simulink model "OutputMVA"  (Simulink 8.7)
settings: Solver=ode45  StartTime=0.0  StopTime=10.0  RelTol=1e-3
undefined symbols (not defined in the file or in its folder): sMP
(part 1 of 3)
settings Model: Creator=rafrey5  LastModifiedBy=hillenb
settings DataIOCC: SignalLoggingSaveFormat=ModelDataLogs
settings OptimizationCC: ExpressionDepthLimit=2147483647
settings DebuggingCC: SolverPrmCheckMsg=warning  FcnCallInpInsideContextMsg=UseLocalSettings  StateNameClashWarn=warning
settings GRTTargetCC: CombineOutputUpdateFcns=off  GRTInterface=on
settings ConfigComp: CovSFcnEnable=off

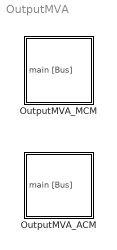
== system OutputMVA ==
  OutputMVA_ACM : Subsystem
      settings: CopyFcn=spsBusSelectorCleanup(gcb,sMP)
  OutputMVA_MCM : Subsystem
      settings: CopyFcn=spsBusSelectorCleanup(gcb,sMP)

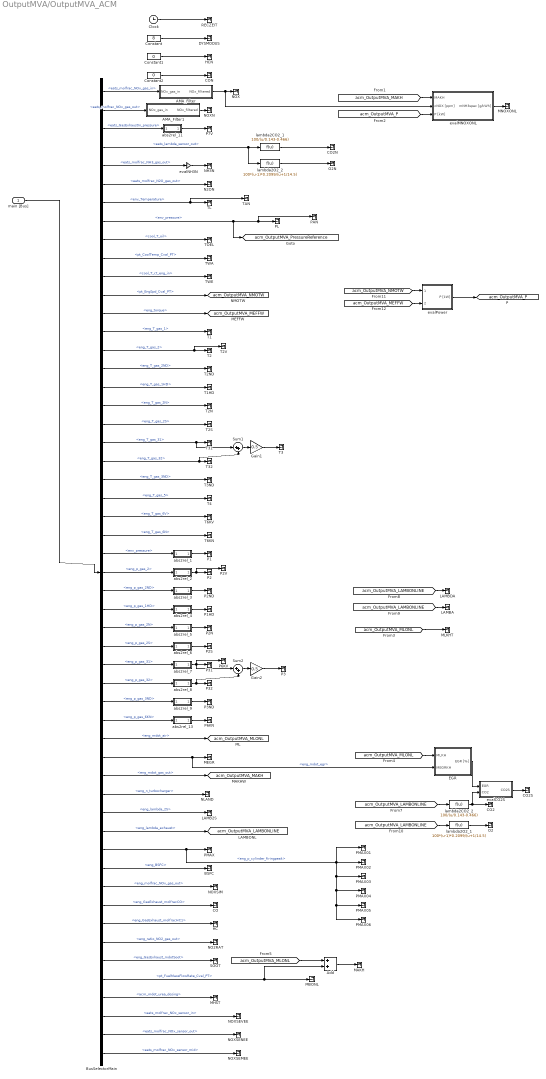
== system OutputMVA/OutputMVA_ACM ==
  main [Bus] : Inport
  AMA_Filter : Subsystem
  AMA_Filter1 : Subsystem
  Add : Sum
  BSFC : Terminator
  BusSelectorMain : BusSelector  OutputSignals=info [Bus].eats_molfrac_NOx_gas_in,info [Bus].eats_molfrac_NOx_gas_out,physics [Bus].eats_GasExhaustIn_pressure,sensor [Bus].eats_lambda_sensor_out,info [Bus].eats_molfrac_NH3_gas_out,info [Bus].eats_molfrac_N2O_gas_out,boundary [Bus].env_Temperature,boundary [Bus].env_pressure,sensor [Bus].cool_T_oil,control [Bus].pt_CoolTemp_Cval_PT,sensor [Bus].cool_T_ct_eng_in,control [Bus].pt_EngSpd_Cval_PT,sensor [Bus].eng_torque,sensor [Bus].eng_T_gas_1,sensor [Bus].eng_T_gas_2,info [Bus].eng_T_gas_2ND,info [Bus].eng_T_gas_1HD,sensor [Bus].eng_T_gas_2N,sensor [Bus].eng_T_gas_2S,sensor [Bus].eng_T_gas_31,sensor [Bus].eng_T_gas_32,info [Bus].eng_T_gas_3ND,info [Bus].eng_T_gas_5,info [Bus].eng_T_gas_6V,sensor [Bus].eng_T_gas_6N,boundary [Bus].env_pressure,info [Bus].eng_p_gas_2,info [Bus].eng_p_gas_2ND,info [Bus].eng_p_gas_1HD,sensor [Bus].eng_p_gas_2N,sensor [Bus].eng_p_gas_2S,sensor [Bus].eng_p_gas_31,info [Bus].eng_p_gas_32,info [Bus].eng_p_gas_3ND,sensor [Bus].eng_p_gas_6KN,sensor [Bus].eng_mdot_air,sensor [Bus].eng_mdot_egr,sensor [Bus].eng_mdot_gas_out,sensor [Bus].eng_n_turbocharger,info [Bus].eng_lambda_2S,sensor [Bus].eng_lambda_exhaust,info [Bus].eng_p_cylinder_firingpeak,info [Bus].eng_BSFC,sensor [Bus].eng_molfrac_NOx_gas_out,physics [Bus].eng_GasExhaust_molfracCO,physics [Bus].eng_GasExhaust_molfracHC1,info [Bus].eng_ratio_NO2_gas_out,physics [Bus].eng_GasExhaust_mdotSoot,control [Bus].pt_FuelMassFlowRate_Cval_PT,actuator [Bus].acm_mdot_urea_dosing,sensor [Bus].eats_molfrac_NOx_sensor_in,sensor [Bus].eats_molfrac_NOx_sensor_out,sensor [Bus].eats_molfrac_NOx_sensor_mid
  CO : Terminator
  CO2 : Terminator
  CO2N : Terminator
  CO2S : Terminator
  CON : Terminator
  Clock : Clock
  Constant : Constant  Value=8
  Constant1 : Constant  Value=0
  Constant2 : Constant  Value=0
  DYSMODUS : Terminator
  EGR : Subsystem
  Gain1 : Gain  Gain=0.5
  Gain2 : Gain  Gain=0.5
  HC : Terminator
  HCN : Terminator
  LAMB2S : Terminator
  LAMBA : Terminator
  LAMBDA : Terminator
  MAKH : Terminator
  MBONL : Terminator
  MEGR : Terminator
  MHST : Terminator
  MLKHT : Terminator
  MNOXONL : Terminator
  N2ON : Terminator
  NH3N : Terminator
  NLAND : Terminator
  NO2RAT : Terminator
  NOX : Terminator
  NOXN : Terminator
  NOXSEMEE : Terminator
  NOXSENEE : Terminator
  NOXSEVEE : Terminator
  NOXSIM : Terminator
  O2 : Terminator
  O2N : Terminator
  P{1..3,31..32} (5 alike) : Terminator
  P1HD : Terminator
  P2N : Terminator
  P2ND : Terminator
  P2S : Terminator
  P2V : Terminator
  P3ND : Terminator
  P6KN : Terminator
  P6KV : Terminator
  P7V : Terminator
  PAN : Terminator
  PL : Terminator
  PMAX : Terminator
  PMAX01 : Terminator
  PMAX02 : Terminator
  PMAX03 : Terminator
  PMAX04 : Terminator
  PMAX05 : Terminator
  PMAX06 : Terminator
  RECZEIT : Terminator
  SOOT : Terminator
  Sum1 : Sum  Inputs=|++
  Sum2 : Sum  Inputs=|++
  T{1..4,31..32} (6 alike) : Terminator
  T1HD : Terminator
  T2N : Terminator
  T2ND : Terminator
  T2S : Terminator
  T2V : Terminator
  T3ND : Terminator
  T6KN : Terminator
  T6KV : Terminator
  TAN : Terminator
  TL : Terminator
  TOEL : Terminator
  TWA : Terminator
  TWE : Terminator
  abs2rel_1 : Subsystem
  abs2rel_11 : Subsystem
  abs2rel_13 : Subsystem
  abs2rel_2 : Subsystem
  abs2rel_3 : Subsystem
  abs2rel_4 : Subsystem
  abs2rel_5 : Subsystem
  abs2rel_6 : Subsystem
  abs2rel_7 : Subsystem
  abs2rel_8 : Subsystem
  abs2rel_9 : Subsystem
  evalCO2S : Subsystem
  evalMNOXONL : Subsystem
  evalNH3N : Gain
  evalPower : Subsystem
  lambda2CO2_1 : Fcn  Expr=100/(u/0.143-0.466)
  lambda2CO2_2 : Fcn  Expr=100/(u/0.143-0.466)
  lambda2O2_1 : Fcn  Expr=100*(u-1)*0.2099/(u+1/14.5)
  lambda2O2_2 : Fcn  Expr=100*(u-1)*0.2099/(u+1/14.5)
  tag scope: acm_OutputMVA_LAMBONLINE=global, acm_OutputMVA_MAKH=global, acm_OutputMVA_MEFFW=global, acm_OutputMVA_MLONL=global, acm_OutputMVA_NMOTW=global, acm_OutputMVA_P=global, acm_OutputMVA_PressureReference=global
  wires:
  [acm_OutputMVA_MLONL] -> Add/1
  Add/1 -> MAKH/1
  BusSelectorMain/49 -> Add/2, MBONL/1  "<pt_FuelMassFlowRate_Cval_PT>"
  BusSelectorMain/50 -> MHST/1  "<acm_mdot_urea_dosing>"
  main [Bus]/1 -> BusSelectorMain/1
  evalNH3N/1 -> NH3N/1
  BusSelectorMain/5 -> evalNH3N/1  "<eats_molfrac_NH3_gas_out>"
  BusSelectorMain/25 -> T6KN/1  "<eng_T_gas_6N>"
  BusSelectorMain/24 -> T6KV/1  "<eng_T_gas_6V>"
  abs2rel_13/1(pressure_relative) -> P6KN/1
  Gain2/1 -> P3/1
  Sum2/1 -> Gain2/1
  Gain1/1 -> T3/1
  Sum1/1 -> Gain1/1
  abs2rel_11/1(pressure_relative) -> P7V/1
  BusSelectorMain/1 -> AMA_Filter/1(NOx_gas_in)  "<eats_molfrac_NOx_gas_in>"
  BusSelectorMain/2 -> AMA_Filter1/1(NOx_gas_in)  "<eats_molfrac_NOx_gas_out>"
  BusSelectorMain/13 -> [acm_OutputMVA_MEFFW]  "<eng_torque>"
  BusSelectorMain/14 -> T1/1  "<eng_T_gas_1>"
  BusSelectorMain/15 -> T2/1, T2V/1  "<eng_T_gas_2>"
  BusSelectorMain/16 -> T2ND/1  "<eng_T_gas_2ND>"
  BusSelectorMain/17 -> T1HD/1  "<eng_T_gas_1HD>"
  BusSelectorMain/18 -> T2N/1  "<eng_T_gas_2N>"
  BusSelectorMain/19 -> T2S/1  "<eng_T_gas_2S>"
  BusSelectorMain/20 -> Sum1/1, T31/1  "<eng_T_gas_31>"
  BusSelectorMain/21 -> Sum1/2, T32/1  "<eng_T_gas_32>"
  BusSelectorMain/22 -> T3ND/1  "<eng_T_gas_3ND>"
  BusSelectorMain/23 -> T4/1  "<eng_T_gas_5>"
  BusSelectorMain/27 -> abs2rel_2/1(pressure_absolute)  "<eng_p_gas_2>"
  BusSelectorMain/7 -> TL/1, TAN/1  "<env_Temperature>"
  BusSelectorMain/8 -> [acm_OutputMVA_PressureReference], PL/1, PAN/1  "<env_pressure>"
  BusSelectorMain/26 -> abs2rel_1/1(pressure_absolute)  "<env_pressure>"
  abs2rel_1/1(pressure_relative) -> P1/1
  abs2rel_2/1(pressure_relative) -> P2/1, P2V/1
  abs2rel_3/1(pressure_relative) -> P2ND/1
  abs2rel_4/1(pressure_relative) -> P1HD/1
  abs2rel_5/1(pressure_relative) -> P2N/1
  abs2rel_6/1(pressure_relative) -> P2S/1
  BusSelectorMain/28 -> abs2rel_3/1(pressure_absolute)  "<eng_p_gas_2ND>"
  BusSelectorMain/29 -> abs2rel_4/1(pressure_absolute)  "<eng_p_gas_1HD>"
  BusSelectorMain/30 -> abs2rel_5/1(pressure_absolute)  "<eng_p_gas_2N>"
  BusSelectorMain/31 -> abs2rel_6/1(pressure_absolute)  "<eng_p_gas_2S>"
  abs2rel_7/1(pressure_relative) -> Sum2/1, P6KV/1, P31/1
  abs2rel_8/1(pressure_relative) -> Sum2/2, P32/1
  abs2rel_9/1(pressure_relative) -> P3ND/1
  BusSelectorMain/37 -> MEGR/1, EGR/2(MEGRKH)  "<eng_mdot_egr>"
  BusSelectorMain/32 -> abs2rel_7/1(pressure_absolute)  "<eng_p_gas_31>"
  BusSelectorMain/33 -> abs2rel_8/1(pressure_absolute)  "<eng_p_gas_32>"
  BusSelectorMain/34 -> abs2rel_9/1(pressure_absolute)  "<eng_p_gas_3ND>"
  BusSelectorMain/35 -> abs2rel_13/1(pressure_absolute)  "<eng_p_gas_6KN>"
  BusSelectorMain/36 -> [acm_OutputMVA_MLONL]  "<eng_mdot_air>"
  BusSelectorMain/38 -> [acm_OutputMVA_MAKH]  "<eng_mdot_gas_out>"
  BusSelectorMain/39 -> NLAND/1  "<eng_n_turbocharger>"
  BusSelectorMain/40 -> LAMB2S/1  "<eng_lambda_2S>"
  BusSelectorMain/41 -> [acm_OutputMVA_LAMBONLINE]  "<eng_lambda_exhaust>"
  BusSelectorMain/42 -> PMAX/1, PMAX02/1, PMAX03/1, PMAX04/1, PMAX05/1, PMAX06/1, PMAX01/1  "<eng_p_cylinder_firingpeak>"
  BusSelectorMain/43 -> BSFC/1  "<eng_BSFC>"
  BusSelectorMain/44 -> NOXSIM/1  "<eng_molfrac_NOx_gas_out>"
  BusSelectorMain/45 -> CO/1  "<eng_GasExhaust_molfracCO>"
  BusSelectorMain/46 -> HC/1  "<eng_GasExhaust_molfracHC1>"
  BusSelectorMain/47 -> NO2RAT/1  "<eng_ratio_NO2_gas_out>"
  BusSelectorMain/48 -> SOOT/1  "<eng_GasExhaust_mdotSoot>"
  lambda2CO2_2/1 -> CO2/1, evalCO2S/2(CO2)
  evalCO2S/1(CO2S) -> CO2S/1
  EGR/1("EGR [%] ") -> evalCO2S/1(EGR)
  Constant/1 -> DYSMODUS/1
  BusSelectorMain/3 -> abs2rel_11/1(pressure_absolute)  "<eats_GasExhaustIn_pressure>"
  BusSelectorMain/12 -> [acm_OutputMVA_NMOTW]  "<pt_EngSpd_Cval_PT>"
  BusSelectorMain/9 -> TOEL/1  "<cool_T_oil>"
  BusSelectorMain/10 -> TWA/1  "<pt_CoolTemp_Cval_PT>"
  BusSelectorMain/11 -> TWE/1  "<cool_T_ct_eng_in>"
  evalPower/1(P [kW]) -> [acm_OutputMVA_P]
  Constant1/1 -> HCN/1
  Constant2/1 -> CON/1
  lambda2CO2_1/1 -> CO2N/1
  BusSelectorMain/4 -> lambda2CO2_1/1, lambda2O2_2/1  "<eats_lambda_sensor_out>"
  [acm_OutputMVA_MAKH] -> evalMNOXONL/1(MAKH)
  evalMNOXONL/1("mNH3spec [g/kWh] ") -> MNOXONL/1
  [acm_OutputMVA_P] -> evalMNOXONL/3(P [kW])
  [acm_OutputMVA_MLONL] -> MLKHT/1
  [acm_OutputMVA_MLONL] -> EGR/1(MLKH)
  [acm_OutputMVA_LAMBONLINE] -> lambda2CO2_2/1
  [acm_OutputMVA_LAMBONLINE] -> LAMBDA/1
  [acm_OutputMVA_LAMBONLINE] -> LAMBA/1
  [acm_OutputMVA_LAMBONLINE] -> lambda2O2_1/1
  lambda2O2_1/1 -> O2/1
  lambda2O2_2/1 -> O2N/1
  [acm_OutputMVA_NMOTW] -> evalPower/1(n [rpm])
  [acm_OutputMVA_MEFFW] -> evalPower/2(M [Nm])
  Clock/1 -> RECZEIT/1
  BusSelectorMain/6 -> N2ON/1  "<eats_molfrac_N2O_gas_out>"
  BusSelectorMain/51 -> NOXSEVEE/1  "<eats_molfrac_NOx_sensor_in>"
  BusSelectorMain/52 -> NOXSENEE/1  "<eats_molfrac_NOx_sensor_out>"
  AMA_Filter/1(NOx_filtered) -> NOX/1, evalMNOXONL/2(cNOX [ppm])
  AMA_Filter1/1(NOx_filtered) -> NOXN/1
  BusSelectorMain/53 -> NOXSEMEE/1  "<eats_molfrac_NOx_sensor_mid>"
